simulink model "zad1"  (R2025b)
settings: Solver=VariableStepAuto  StartTime=0.0  StopTime=3500  RelTol=1e-3
libraries: fuzblock x2
settings Model: Creator=jovan  LastModifiedBy=Katarina

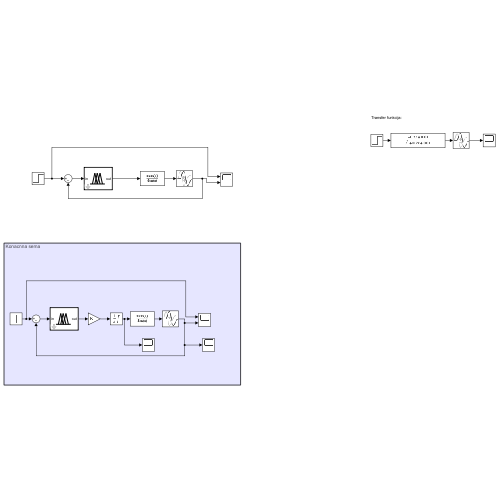
[thumbnail: Simulink's stored preview of the top-level diagram]
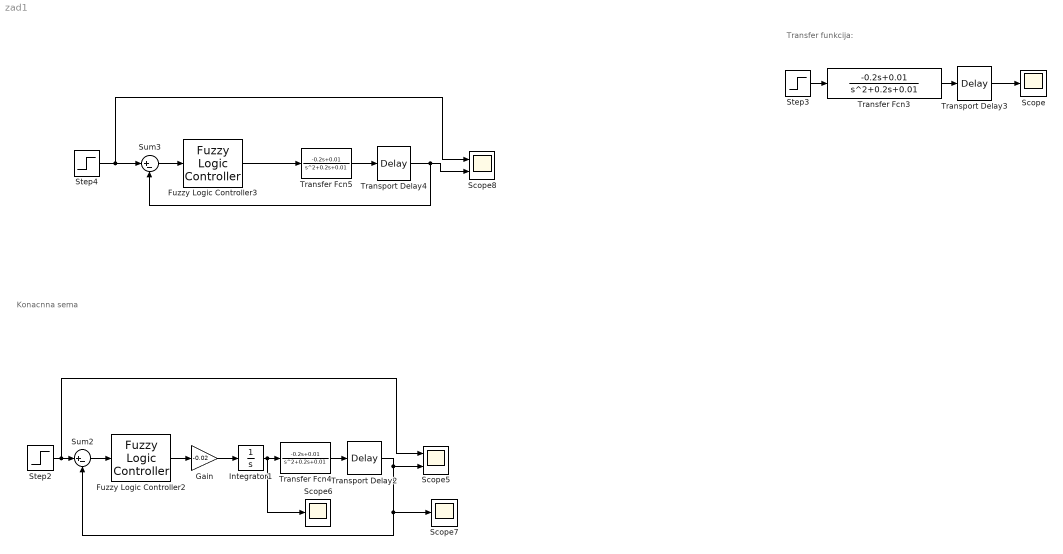
== system zad1 ==
  note: Konacnna sema
  note: Transfer funkcija:
  Fuzzy Logic Controller2 : fuzblock/Fuzzy Logic  Controller  FIS='kontrolaBrzine.fis'  OutputSampleNumber=101  DataType=double  UseLookupTable=off  NumBreakpoints=10  FuzzifiedInputs=off  RuleFiringStrengths=off  RuleOutputs=off  AggregatedOutputs=off  SimulateUsing=Interpreted execution  OutOfRangeInputValueMessage=warning  NoRuleFiredMessage=warning  EmptyOutputFuzzySetMessage=warning
  Fuzzy Logic Controller3 : fuzblock/Fuzzy Logic  Controller  FIS='kontrolaBrzine.fis'  OutputSampleNumber=101  DataType=double  UseLookupTable=off  NumBreakpoints=10  FuzzifiedInputs=off  RuleFiringStrengths=off  RuleOutputs=off  AggregatedOutputs=off  SimulateUsing=Interpreted execution  OutOfRangeInputValueMessage=warning  NoRuleFiredMessage=warning  EmptyOutputFuzzySetMessage=warning
  Gain : Gain  Gain=-0.02
  Integrator1 : Integrator  LimitOutput=on  UpperSaturationLimit=1.5  LowerSaturationLimit=-1.5
  Scope : Scope
      settings: ActiveDisplayYMinimum=-1  ActiveDisplayYMaximum=1
  Scope5 : Scope  NumInputPorts=2
      settings: ActiveDisplayYMinimum=-3.4700005227922581  ActiveDisplayYMaximum=2.3442666414567404  DataLoggingVariableName=ScopeData5
  Scope6 : Scope
      settings: ActiveDisplayYMinimum=-4.9366047496322016  ActiveDisplayYMaximum=5.1764412247857532  DataLoggingVariableName=ScopeData6
  Scope7 : Scope
      settings: ActiveDisplayYMinimum=-1  ActiveDisplayYMaximum=1  DataLoggingVariableName=ScopeData7
  Scope8 : Scope  NumInputPorts=2
      settings: ActiveDisplayYMinimum=-2.3323485682731588  ActiveDisplayYMaximum=6.6259996978809141  DataLoggingVariableName=ScopeData8
  Step2 : Step  Time=1100  Before=-1  SampleTime=0
  Step3 : Step  Time=1100  Before=-1  SampleTime=0
  Step4 : Step  Time=1100  Before=-1  SampleTime=0
  Sum2 : Sum  Inputs=|+-
  Sum3 : Sum  Inputs=|+-
  Transfer Fcn3 : TransferFcn  Numerator=[-0.2 0.01]  Denominator=[1 0.2 0.01]
  Transfer Fcn4 : TransferFcn  Numerator=[-0.2 0.01]  Denominator=[1 0.2 0.01]
  Transfer Fcn5 : TransferFcn  Numerator=[-0.2 0.01]  Denominator=[1 0.2 0.01]
  Transport Delay2 : TransportDelay  DelayTime=4
  Transport Delay3 : TransportDelay  DelayTime=4
  Transport Delay4 : TransportDelay  DelayTime=4
  wires:
  Step3/1 -> Transfer Fcn3/1
  Transfer Fcn3/1 -> Transport Delay3/1
  Transport Delay3/1 -> Scope/1
  Transfer Fcn4/1 -> Transport Delay2/1
  Integrator1/1 -> Scope6/1, Transfer Fcn4/1
  Transport Delay2/1 -> Scope5/2, Scope7/1, Sum2/2
  Sum2/1 -> Fuzzy Logic Controller2/1
  Step2/1 -> Scope5/1, Sum2/1
  Fuzzy Logic Controller2/1 -> Gain/1
  Gain/1 -> Integrator1/1
  Step4/1 -> Sum3/1, Scope8/1
  Transfer Fcn5/1 -> Transport Delay4/1
  Fuzzy Logic Controller3/1 -> Transfer Fcn5/1
  Sum3/1 -> Fuzzy Logic Controller3/1
  Transport Delay4/1 -> Scope8/2, Sum3/2
